simulink model "kadai_2_1"  (R2018a)
settings: Solver=VariableStepAuto  StartTime=0.0  StopTime=inf  RelTol=1e-3
undefined symbols (not defined in the file or in its folder): Angular, Linear
libraries: robotlib x7
settings Model: Creator=admin  LastModifiedBy=admin

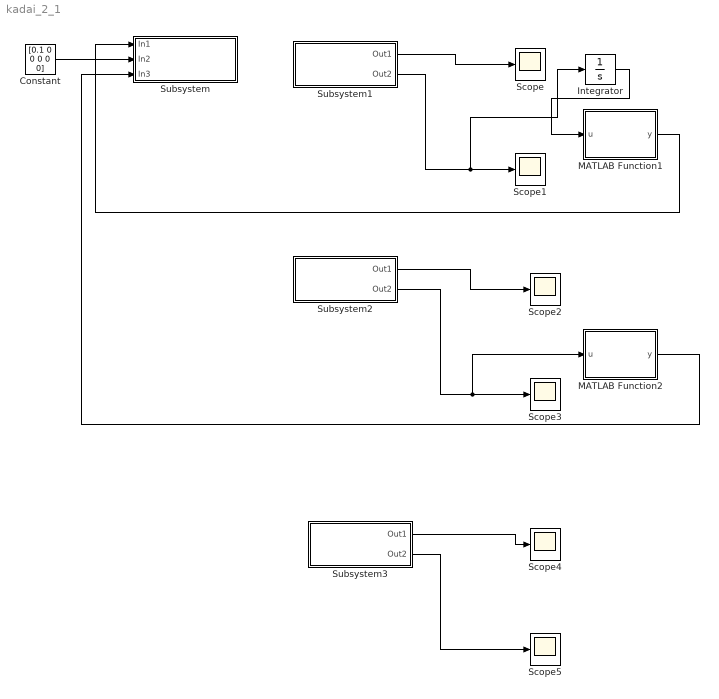
== system kadai_2_1 ==
  Constant : Constant  Value="[0.1 0 0  0 0 0]"
  Integrator : Integrator
  MATLAB Function1 : MATLAB Function  TreatAsAtomicUnit=on
  MATLAB Function2 : MATLAB Function  TreatAsAtomicUnit=on
  Scope{,1..5} (6 alike) : Scope
  Subsystem : Subsystem
  Subsystem1 : Subsystem
  Subsystem2 : Subsystem
  Subsystem3 : Subsystem
  wires:
  Constant/1 -> Subsystem/1(In1)
  Subsystem1/1(Out1) -> Scope/1
  Subsystem1/2(Out2) -> Integrator/1, Scope1/1
  Subsystem2/2(Out2) -> MATLAB Function2/1(u), Scope3/1
  Subsystem2/1(Out1) -> Scope2/1
  Subsystem3/2(Out2) -> Scope5/1
  Subsystem3/1(Out1) -> Scope4/1
  MATLAB Function1/1(y) -> Subsystem/2(In2)
  MATLAB Function2/1(y) -> Subsystem/3(In3)
  Integrator/1 -> MATLAB Function1/1(u)

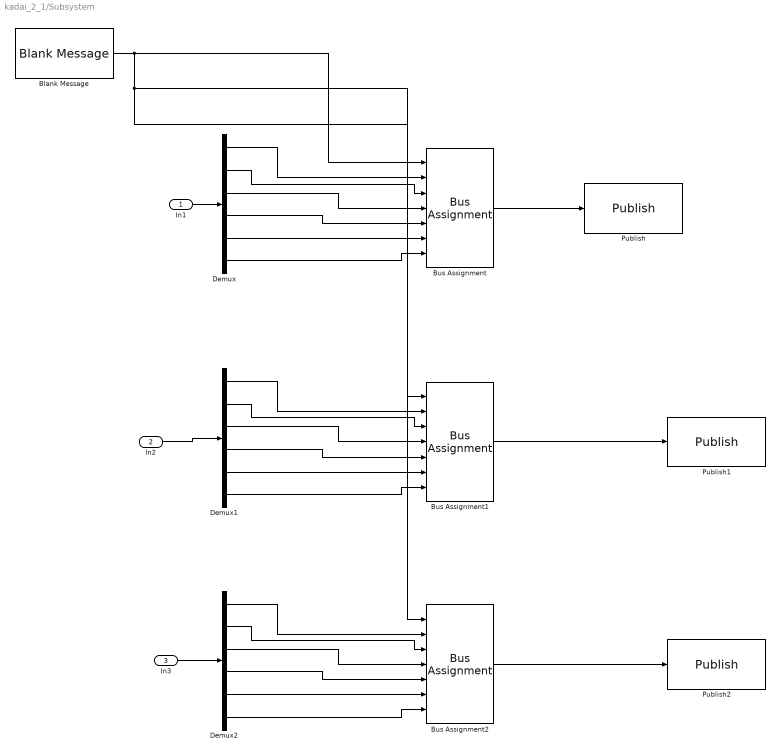
== system kadai_2_1/Subsystem ==
  In1 : Inport
  In2 : Inport  Port=2
  In3 : Inport  Port=3
  Blank Message : robotlib/Blank Message  SourceLibraryInfo=This block requires Robotics System Toolbox  messageType=geometry_msgs/Twist  SampleTime=inf
      settings: SourceProductBaseCode=RO
  Bus Assignment : BusAssignment  AssignedSignals=Linear.X,Linear.Y,Linear.Z,Angular.X,Angular.Y,Angular.Z
  Bus Assignment1 : BusAssignment  AssignedSignals=Linear.X,Linear.Y,Linear.Z,Angular.X,Angular.Y,Angular.Z
  Bus Assignment2 : BusAssignment  AssignedSignals=Linear.X,Linear.Y,Linear.Z,Angular.X,Angular.Y,Angular.Z
  Demux : Demux  Outputs=6
  Demux1 : Demux  Outputs=6
  Demux2 : Demux  Outputs=6
  Publish : robotlib/Publish  SourceLibraryInfo=This block requires Robotics System Toolbox  topicSource=Specify your own  topic=/cmd_vel  messageType=geometry_msgs/Twist  messageQueueLength=1
      settings: SourceProductBaseCode=RO
  Publish1 : robotlib/Publish  SourceLibraryInfo=This block requires Robotics System Toolbox  topicSource=Specify your own  topic=/cmd_vel  messageType=geometry_msgs/Twist  messageQueueLength=1
      settings: SourceProductBaseCode=RO
  Publish2 : robotlib/Publish  SourceLibraryInfo=This block requires Robotics System Toolbox  topicSource=Specify your own  topic=/cmd_vel  messageType=geometry_msgs/Twist  messageQueueLength=1
      settings: SourceProductBaseCode=RO
  wires:
  In1/1 -> Demux/1
  Demux/1 -> Bus Assignment/2
  Demux/2 -> Bus Assignment/3
  Demux/3 -> Bus Assignment/4
  Demux/4 -> Bus Assignment/5
  Demux/5 -> Bus Assignment/6
  Demux/6 -> Bus Assignment/7
  Bus Assignment/1 -> Publish/1
  Demux1/1 -> Bus Assignment1/2
  Demux1/3 -> Bus Assignment1/4
  Demux1/2 -> Bus Assignment1/3
  Demux1/4 -> Bus Assignment1/5
  Demux1/5 -> Bus Assignment1/6
  Demux1/6 -> Bus Assignment1/7
  In2/1 -> Demux1/1
  Bus Assignment1/1 -> Publish1/1
  Blank Message/1 -> Bus Assignment2/1, Bus Assignment1/1, Bus Assignment/1
  Bus Assignment2/1 -> Publish2/1
  Demux2/5 -> Bus Assignment2/6
  Demux2/4 -> Bus Assignment2/5
  Demux2/3 -> Bus Assignment2/4
  Demux2/6 -> Bus Assignment2/7
  Demux2/2 -> Bus Assignment2/3
  Demux2/1 -> Bus Assignment2/2
  In3/1 -> Demux2/1

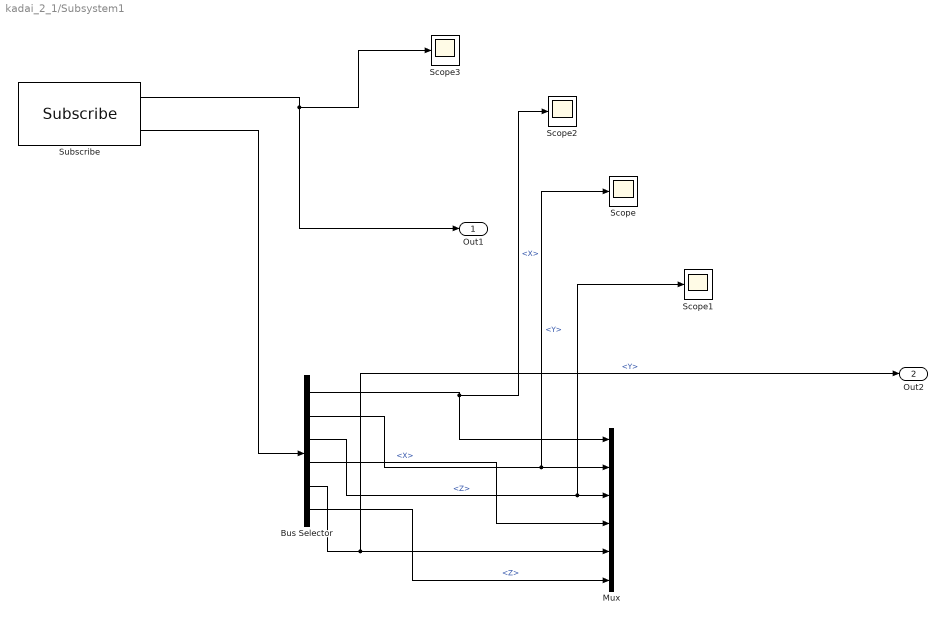
== system kadai_2_1/Subsystem1 ==
  Bus Selector : BusSelector  OutputSignals=LinearAcceleration.X,LinearAcceleration.Y,LinearAcceleration.Z,AngularVelocity.X,AngularVelocity.Y,AngularVelocity.Z
  Mux : Mux  Inputs=6
  Scope{,1..3} (4 alike) : Scope
  Subscribe : robotlib/Subscribe  SourceLibraryInfo=This block requires Robotics System Toolbox  topicSource=Select from ROS network  topic=/imu  messageType=sensor_msgs/Imu  sampleTime=0.1  messageQueueLength=1
      settings: SourceProductBaseCode=RO
  Out1 : Outport
  Out2 : Outport  Port=2
  wires:
  Subscribe/1 -> Scope3/1, Out1/1
  Subscribe/2 -> Bus Selector/1
  Bus Selector/1 -> Scope2/1, Mux/1  "<X>"
  Bus Selector/2 -> Scope/1, Mux/2  "<Y>"
  Bus Selector/3 -> Scope1/1, Mux/3  "<Z>"
  Bus Selector/4 -> Mux/4  "<X>"
  Bus Selector/5 -> Out2/1, Mux/5  "<Y>"
  Bus Selector/6 -> Mux/6  "<Z>"

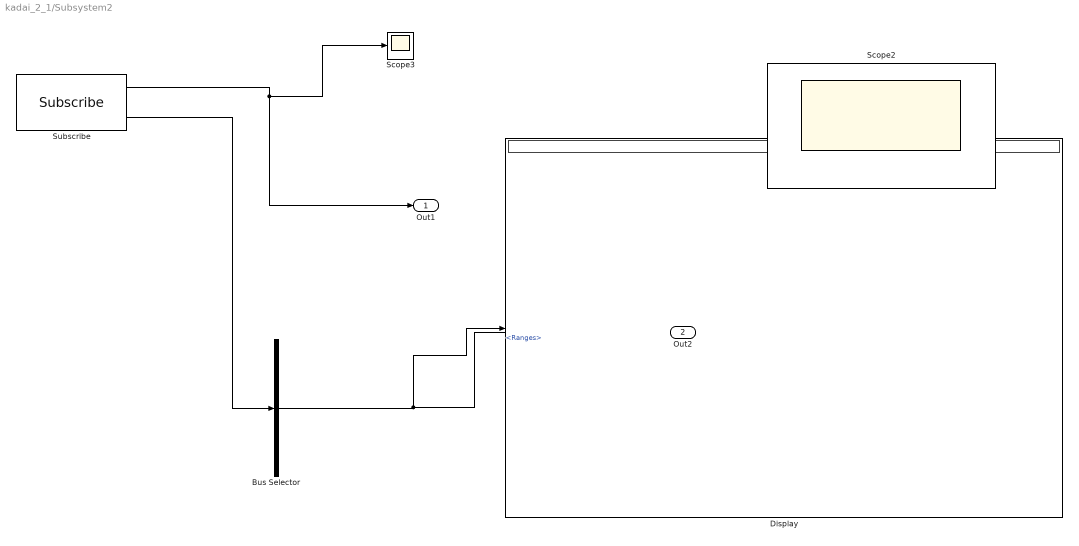
== system kadai_2_1/Subsystem2 ==
  Bus Selector : BusSelector  OutputSignals=Ranges
  Display : Display
  Scope2 : Scope
  Scope3 : Scope
  Subscribe : robotlib/Subscribe  SourceLibraryInfo=This block requires Robotics System Toolbox  topicSource=Select from ROS network  topic=/scan  messageType=sensor_msgs/LaserScan  sampleTime=0.1  messageQueueLength=1
      settings: SourceProductBaseCode=RO
  Out1 : Outport
  Out2 : Outport  Port=2
  wires:
  Subscribe/1 -> Scope3/1, Out1/1
  Subscribe/2 -> Bus Selector/1
  Bus Selector/1 -> Display/1, Out2/1  "<Ranges>"

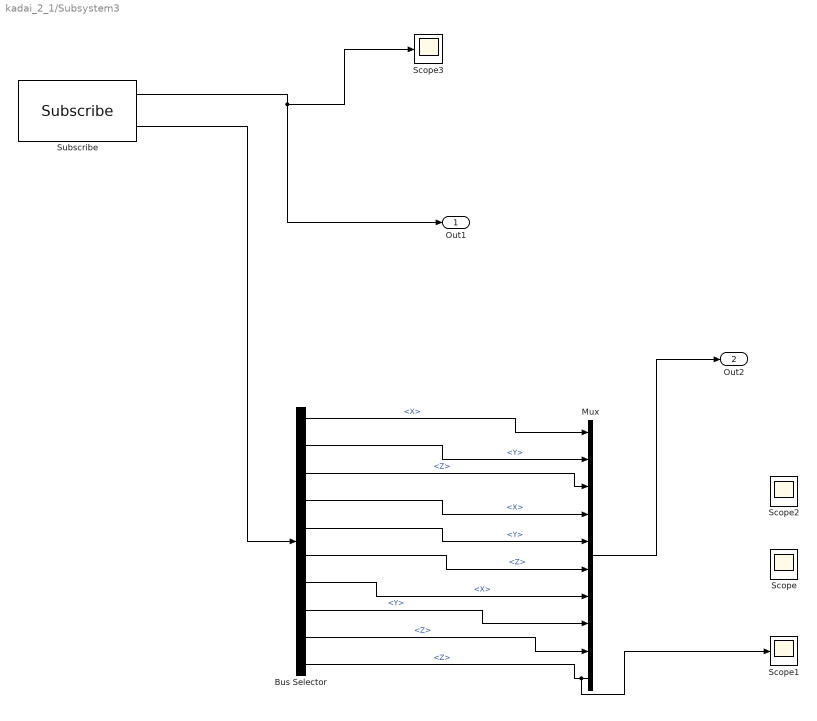
== system kadai_2_1/Subsystem3 ==
  Bus Selector : BusSelector  OutputSignals=Pose.Pose.Position.X,Pose.Pose.Position.Y,Pose.Pose.Position.Z,Pose.Pose.Orientation.X,Pose.Pose.Orientation.Y,Pose.Pose.Orientation.Z,Twist.Twist.Linear.X,Twist.Twist.Linear.Y,Twist.Twist.Linear.Z,Twist.Twist.Angular.Z
  Mux : Mux  Inputs=10
  Scope{,1..3} (4 alike) : Scope
  Subscribe : robotlib/Subscribe  SourceLibraryInfo=This block requires Robotics System Toolbox  topicSource=Select from ROS network  topic=/odom  messageType=nav_msgs/Odometry  sampleTime=0.1  messageQueueLength=1
      settings: SourceProductBaseCode=RO
  Out1 : Outport
  Out2 : Outport  Port=2
  wires:
  Subscribe/1 -> Scope3/1, Out1/1
  Subscribe/2 -> Bus Selector/1
  Mux/1 -> Out2/1
  Bus Selector/1 -> Mux/1  "<X>"
  Bus Selector/2 -> Mux/2  "<Y>"
  Bus Selector/3 -> Mux/3  "<Z>"
  Bus Selector/4 -> Mux/4  "<X>"
  Bus Selector/5 -> Mux/5  "<Y>"
  Bus Selector/6 -> Mux/6  "<Z>"
  Bus Selector/7 -> Mux/7  "<X>"
  Bus Selector/8 -> Mux/8  "<Y>"
  Bus Selector/9 -> Mux/9  "<Z>"
  Bus Selector/10 -> Scope1/1  "<Z>"

== matlab function kadai_2_1/MATLAB Function1 ==
  data: u input; y output
function y = fcn(u)
if u < -0.3
    y = [0.2 0 0 0 0 0];
else 
    y=[0.1 0 0  0 0 0];
end
%y = u;

== matlab function kadai_2_1/MATLAB Function2 ==
  data: u input; y output
function y = fcn(u)
disp(u)
if u(1) < 1
    y = [0 0 0 0 0 0];
else 
    y=[0.1 0 0  0 0 0];
end
%y = u;
